simulink model "MYDM2"  (R2021a)
settings: Solver=VariableStepAuto  StartTime=0.0  StopTime=12  RelTol=1e-3
libraries: dspvision x4, dsparch4 x2, dspquant2 x2
settings Model: Creator=RUKU  LastModifiedBy=RUKU

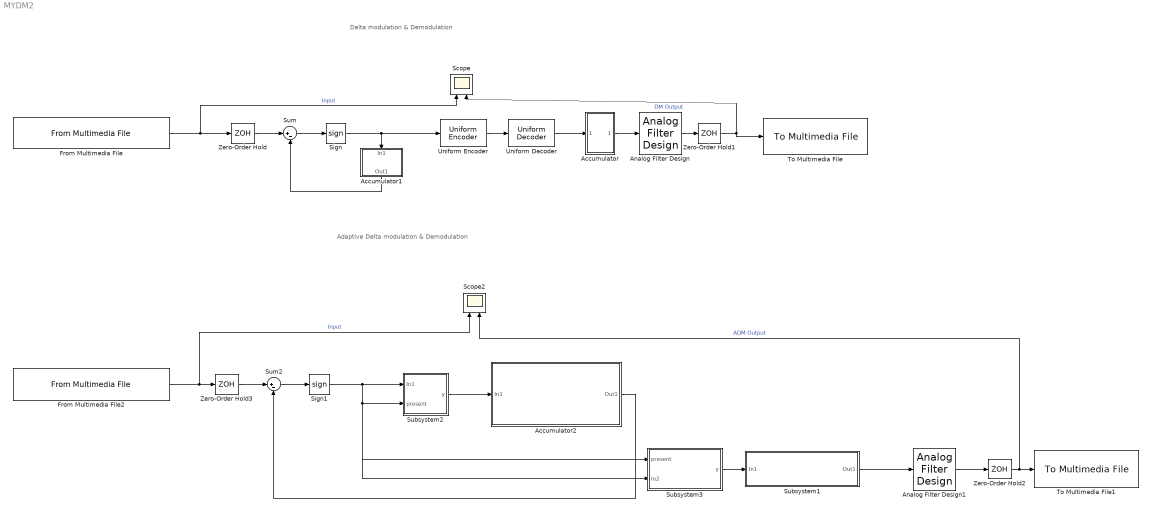
== system MYDM2 ==
  note: Delta modulation & Demodulation
  note: Adaptive Delta modulation & Demodulation
  Accumulator : Subsystem
  Accumulator1 : Subsystem
  Accumulator2 : Subsystem
  Analog Filter Design : dsparch4/Analog Filter Design  method=Butterworth  filttype=Lowpass  N=8  Wlo=2*pi*600  Whi=80  Rp=2  Rs=40
  Analog Filter Design1 : dsparch4/Analog Filter Design  method=Butterworth  filttype=Lowpass  N=8  Wlo=2*pi*1000  Whi=80  Rp=2  Rs=40
  From Multimedia File : dspvision/From Multimedia File  inputFilename=D:\Yekra\OneDrive - BUET\MatLab works\DSP Lab Test1\Speech 1-10 Rakib.mp3  readRange=[1 Inf]  loop=on  numPlays=1  outputStreams=Audio only  videoDataType=single  audioDataType=double  inheritSampleTime=on  userDefinedSampleTime=1/30  noAudioOutput=off  isIntensityVideo=off  fourcc=RGB  colorVideoFormat=Separate color signals  outputEOF=off  dataOrg=Column-major  audioFrameSize=1  computeAudioFrameSize=off  outSamplingMode=Sample based
  From Multimedia File2 : dspvision/From Multimedia File  inputFilename=D:\Yekra\OneDrive - BUET\MatLab works\DSP Lab Test1\Speech 1-10 Rakib.mp3  readRange=[1 Inf]  loop=on  numPlays=1  outputStreams=Audio only  videoDataType=single  audioDataType=double  inheritSampleTime=on  userDefinedSampleTime=1/30  noAudioOutput=off  isIntensityVideo=off  fourcc=RGB  colorVideoFormat=Separate color signals  outputEOF=off  dataOrg=Column-major  audioFrameSize=1  computeAudioFrameSize=off  outSamplingMode=Sample based
  Scope : Scope  NumInputPorts=2
  Scope2 : Scope  NumInputPorts=2
  Sign : Signum
  Sign1 : Signum
  Subsystem1 : Subsystem
  Subsystem2 : Subsystem
  Subsystem3 : Subsystem
  Sum : Sum  Inputs=|+-
  Sum2 : Sum  Inputs=|+-
  To Multimedia File : dspvision/To Multimedia File  outputFilename=DM_output.wav  streamSelection=Audio only  videoCompressor=None (uncompressed)  audioCompressor=None (uncompressed)  imagePorts=Separate color signals  fileType=WAV  audioDatatype=16-bit integer  fourcc=RGB  videoQuality=75  mj2000CompFactor=10
  To Multimedia File1 : dspvision/To Multimedia File  outputFilename=ADM_output.wav  streamSelection=Audio only  videoCompressor=None (uncompressed)  audioCompressor=None (uncompressed)  imagePorts=Separate color signals  fileType=WAV  audioDatatype=16-bit integer  fourcc=RGB  videoQuality=75  mj2000CompFactor=10
  Uniform Decoder : dspquant2/Uniform Decoder  peak=2  bits=16  overflowMode=Saturate  otype=Double
      settings: SourceProductBaseCode=DS
  Uniform Encoder : dspquant2/Uniform Encoder  peak=2  bits=16  otype=Signed integer
  Zero-Order Hold{,1..3} (4 alike) : ZeroOrderHold  SampleTime=1/16000
  wires:
  Zero-Order Hold/1 -> Sum/1
  Sum/1 -> Sign/1
  Sign/1 -> Uniform Encoder/1, Accumulator1/1(In1)
  From Multimedia File/1 -> Scope/1, Zero-Order Hold/1  "Input"
  Analog Filter Design/1 -> Zero-Order Hold1/1
  Zero-Order Hold1/1 -> To Multimedia File/1, Scope/2  "DM Output"
  Accumulator/1(Out1) -> Analog Filter Design/1
  Accumulator1/1(Out1) -> Sum/2
  Uniform Encoder/1 -> Uniform Decoder/1
  Uniform Decoder/1 -> Accumulator/1(In1)
  Subsystem1/1(Out1) -> Analog Filter Design1/1
  Subsystem3/1(y) -> Subsystem1/1(In1)
  From Multimedia File2/1 -> Scope2/1, Zero-Order Hold3/1  "Input"
  Sum2/1 -> Sign1/1
  Sign1/1 -> Subsystem2/1(In1), Subsystem3/1(present), Subsystem2/2(present), Subsystem3/2(In2)
  Subsystem2/1(y) -> Accumulator2/1(In1)
  Zero-Order Hold3/1 -> Sum2/1
  Accumulator2/1(Out1) -> Sum2/2
  Analog Filter Design1/1 -> Zero-Order Hold2/1
  Zero-Order Hold2/1 -> Scope2/2, To Multimedia File1/1  "ADM Output"

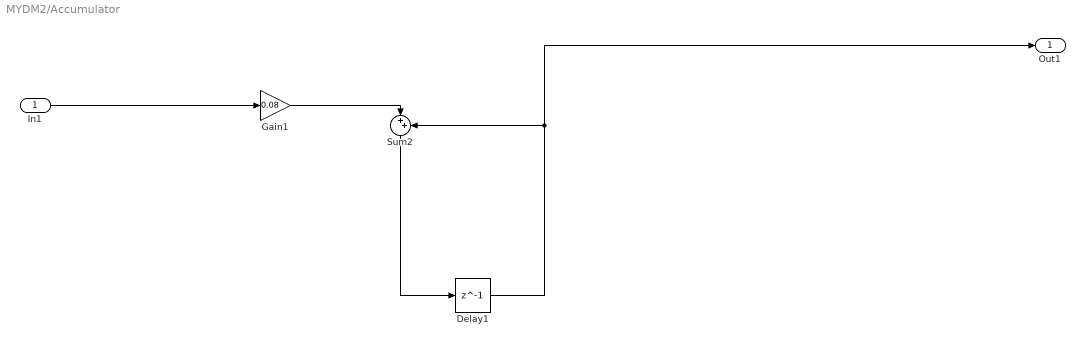
== system MYDM2/Accumulator ==
  In1 : Inport
  Delay1 : Delay  DelayLength=1
  Gain1 : Gain  Gain=0.08
  Sum2 : Sum  Inputs=|++
  Out1 : Outport
  wires:
  In1/1 -> Gain1/1
  Delay1/1 -> Out1/1, Sum2/2
  Sum2/1 -> Delay1/1
  Gain1/1 -> Sum2/1

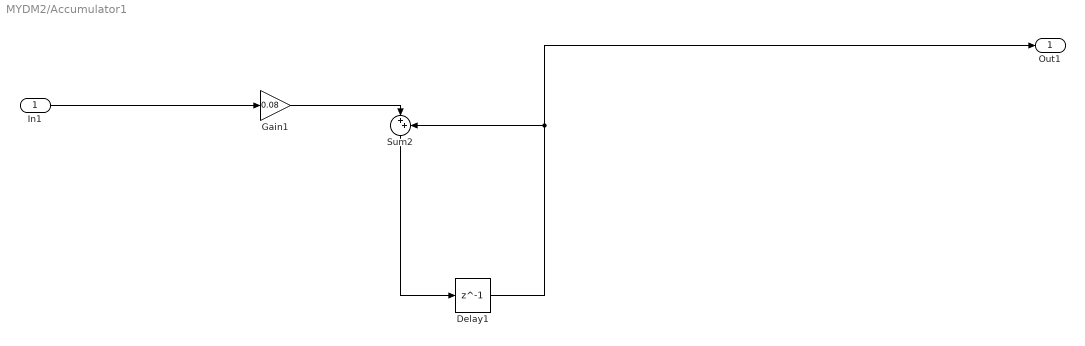
== system MYDM2/Accumulator1 ==
  In1 : Inport
  Delay1 : Delay  DelayLength=1
  Gain1 : Gain  Gain=0.08
  Sum2 : Sum  Inputs=|++
  Out1 : Outport
  wires:
  In1/1 -> Gain1/1
  Delay1/1 -> Out1/1, Sum2/2
  Sum2/1 -> Delay1/1
  Gain1/1 -> Sum2/1

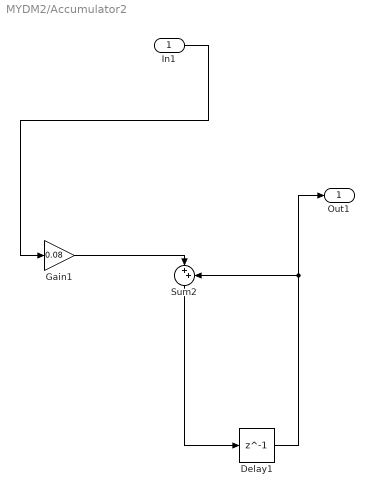
== system MYDM2/Accumulator2 ==
  In1 : Inport
  Delay1 : Delay  DelayLength=1
  Gain1 : Gain  Gain=0.08
  Sum2 : Sum  Inputs=|++
  Out1 : Outport
  wires:
  Delay1/1 -> Out1/1, Sum2/2
  Gain1/1 -> Sum2/1
  Sum2/1 -> Delay1/1
  In1/1 -> Gain1/1

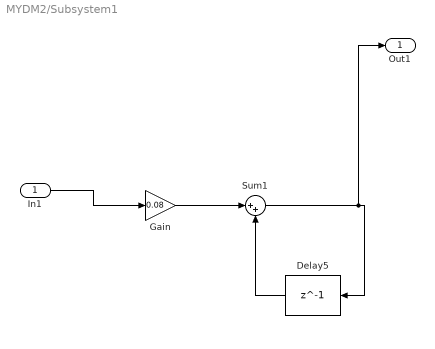
== system MYDM2/Subsystem1 ==
  In1 : Inport
  Delay5 : Delay  DelayLength=1  InputProcessing=Columns as channels (frame based)
  Gain : Gain  Gain=0.08
  Sum1 : Sum  Inputs=|++
  Out1 : Outport
  wires:
  Delay5/1 -> Sum1/2
  Sum1/1 -> Out1/1, Delay5/1
  Gain/1 -> Sum1/1
  In1/1 -> Gain/1

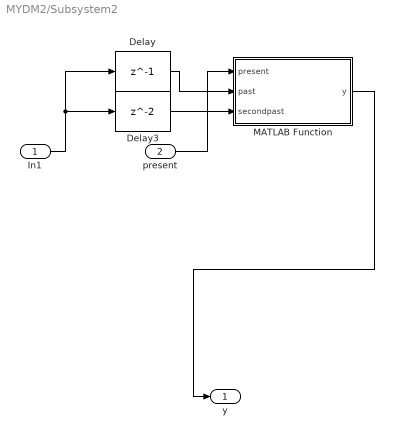
== system MYDM2/Subsystem2 ==
  In1 : Inport
  present : Inport  Port=2
  Delay : Delay  DelayLength=1  InputProcessing=Columns as channels (frame based)
  Delay3 : Delay  InputProcessing=Columns as channels (frame based)
  MATLAB Function : MATLAB Function  TreatAsAtomicUnit=on
  y : Outport
  wires:
  In1/1 -> Delay3/1, Delay/1
  present/1 -> MATLAB Function/1(present)
  Delay3/1 -> MATLAB Function/3(secondpast)
  Delay/1 -> MATLAB Function/2(past)
  MATLAB Function/1(y) -> y/1

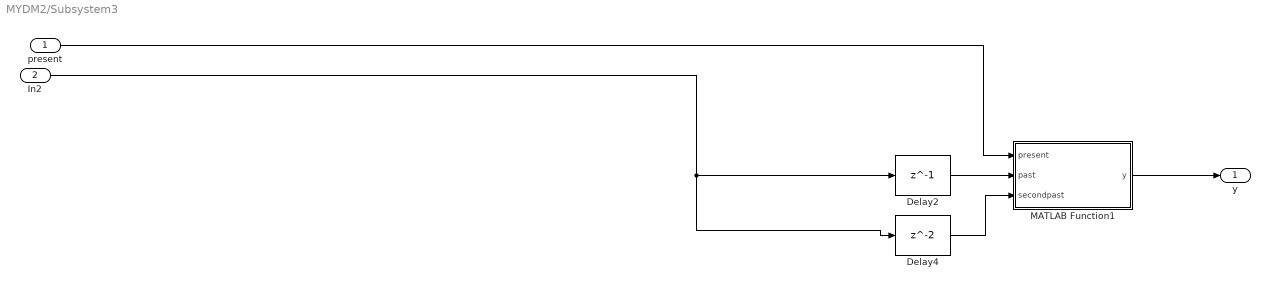
== system MYDM2/Subsystem3 ==
  present : Inport
  In2 : Inport  Port=2
  Delay2 : Delay  DelayLength=1  InputProcessing=Columns as channels (frame based)
  Delay4 : Delay  InputProcessing=Columns as channels (frame based)
  MATLAB Function1 : MATLAB Function  TreatAsAtomicUnit=on
  y : Outport
  wires:
  present/1 -> MATLAB Function1/1(present)
  Delay2/1 -> MATLAB Function1/2(past)
  In2/1 -> Delay4/1, Delay2/1
  MATLAB Function1/1(y) -> y/1
  Delay4/1 -> MATLAB Function1/3(secondpast)

== matlab function MYDM2/Subsystem2/MATLAB Function ==
  data: present input; y output; past input; secondpast input
function y = control(present,past,secondpast)

if present == past 
    if present == secondpast
        y=4*present;
    else
        y=2*present;
    end
else
    y=1*present;
    
end
end

== matlab function MYDM2/Subsystem3/MATLAB Function1 ==
  data: present input; y output; past input; secondpast input
function y = control(present,past,secondpast)

if present == past 
    if present == secondpast
        y=4*present;
    else
        y=2*present;
    end
else
    y=1*present;
    
end
end
